simulink model "uklad3"  (R2023a)
settings: Solver=VariableStepAuto  StartTime=0.0  StopTime=300  RelTol=1e-3
undefined symbols (not defined in the file): k1, k2, kr, T1, T2, tau, Td, Ti, Tp
settings Model: Creator=jpawl  LastModifiedBy=jpawl

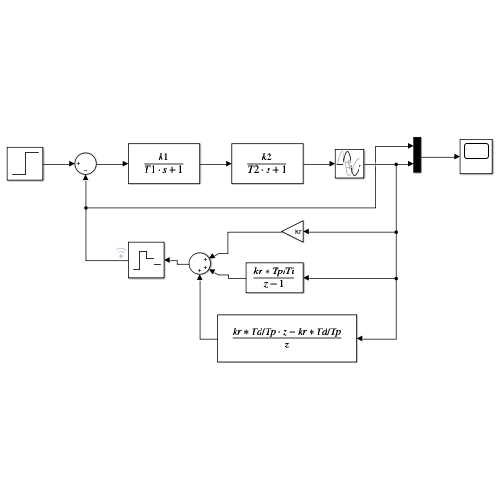
[thumbnail: Simulink's stored preview of the top-level diagram]
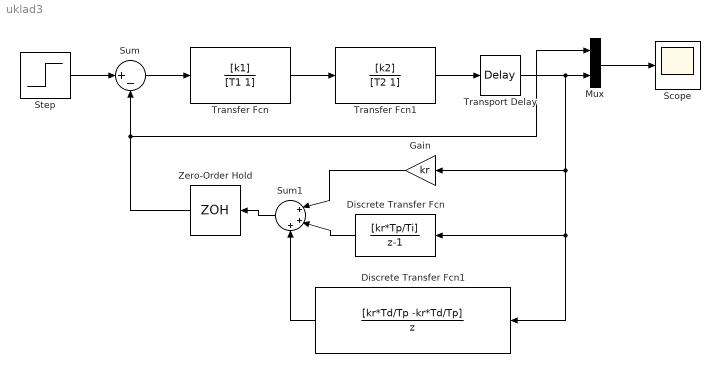
== system uklad3 ==
  Discrete Transfer Fcn : DiscreteTransferFcn  Numerator=[kr*Tp/Ti]  Denominator=[1 -1]
  Discrete Transfer Fcn1 : DiscreteTransferFcn  Numerator=[kr*Td/Tp -kr*Td/Tp]  Denominator=[1 0]
  Gain : Gain  Gain=kr
  Mux : Mux  Inputs=2
  Scope : Scope
  Step : Step  SampleTime=Tp
  Sum : Sum  Inputs=|+-
  Sum1 : Sum  Inputs=|+++
  Transfer Fcn : TransferFcn  Numerator=[k1]  Denominator=[T1 1]
  Transfer Fcn1 : TransferFcn  Numerator=[k2]  Denominator=[T2 1]
  Transport Delay : TransportDelay  DelayTime=-tau
  Zero-Order Hold : ZeroOrderHold  SampleTime=Tp
  wires:
  Step/1 -> Sum/1
  Sum/1 -> Transfer Fcn/1
  Transfer Fcn/1 -> Transfer Fcn1/1
  Transfer Fcn1/1 -> Transport Delay/1
  Zero-Order Hold/1 -> Mux/1, Sum/2
  Sum1/1 -> Zero-Order Hold/1
  Gain/1 -> Sum1/1
  Discrete Transfer Fcn/1 -> Sum1/2
  Discrete Transfer Fcn1/1 -> Sum1/3
  Transport Delay/1 -> Gain/1, Discrete Transfer Fcn/1, Discrete Transfer Fcn1/1, Mux/2
  Mux/1 -> Scope/1
